simulink model "DCmotor_block"  (R2014b)
settings: Solver=ode23t  StartTime=0.0  StopTime=10  MaxStep=0.01  RelTol=1e-3
values from neighbouring files (symbols this model uses):
  Cv = 1.3*10^(-3) *10^(-3)*60/(2*pi)    (= 1.24140855612e-05)    [load_values.m]    (also in task6.m)
  J = 60 * 10^(-3) *10^(-4)    (= 6e-06)    [load_values.m]    (also in task6.m)
  kE = 4.555 *10^(-3)*60/(2*pi)    (= 0.043497045947)    [load_values.m]    (also in task6.m)
  kM = 43.5*10^(-3)    (= 0.0435)    [load_values.m]    (also in task6.m)
  L = [24.5, 19.6, 13.9, 13.1, 7   ] *10^(-3)    [load_values.m]    (also in task6.m = 0.00011)
  R = 1.45    [load_values.m]    (also in task6.m)
undefined symbols (not defined in the file or in its folder): MH
settings Model: Creator=Davide  LastModifiedBy=davidebo
settings DebuggingCC: SolverPrmCheckMsg=none

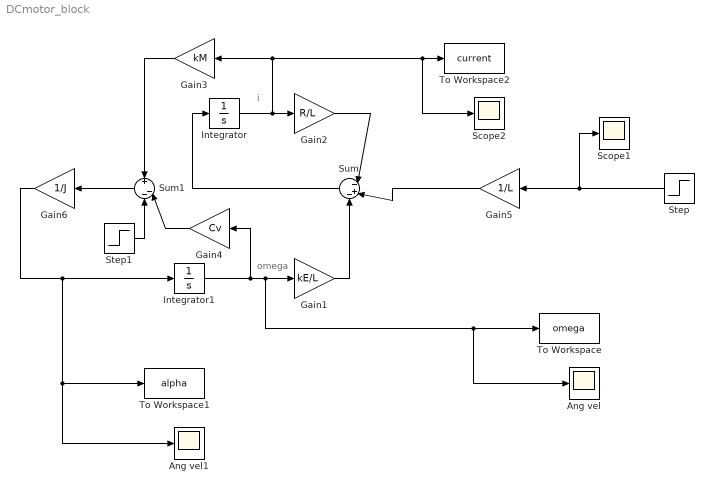
== system DCmotor_block ==
  note: omega
  note: i
  Ang vel : Scope
      settings: TimeRange=10
  Ang vel1 : Scope
      settings: TimeRange=10  SaveName=ScopeData2
  Gain1 : Gain  Gain=kE/L
  Gain2 : Gain  Gain=R/L
  Gain3 : Gain  Gain=kM
  Gain4 : Gain  Gain=Cv
  Gain5 : Gain  Gain=1/L
  Gain6 : Gain  Gain=1/J
  Integrator : Integrator
  Integrator1 : Integrator
  Scope1 : Scope
      settings: TimeRange=10
  Scope2 : Scope
      settings: TimeRange=10  SaveName=ScopeData3
  Step : Step  After=24  SampleTime=0
  Step1 : Step  Time=2  After=MH  SampleTime=0
  Sum : Sum  Inputs=|-+-
  Sum1 : Sum  Inputs=+|--
  To Workspace : ToWorkspace  VariableName=omega  SaveFormat=Timeseries  SampleTime=-1
  To Workspace1 : ToWorkspace  VariableName=alpha  SaveFormat=Timeseries  SampleTime=-1
  To Workspace2 : ToWorkspace  VariableName=current  SaveFormat=Timeseries  SampleTime=-1
  wires:
  Integrator/1 -> Scope2/1, To Workspace2/1, Gain3/1, Gain2/1
  Integrator1/1 -> Gain4/1, Ang vel/1, To Workspace/1, Gain1/1
  Gain2/1 -> Sum/1
  Sum/1 -> Integrator/1
  Gain1/1 -> Sum/3
  Gain3/1 -> Sum1/1
  Gain4/1 -> Sum1/2
  Gain5/1 -> Sum/2
  Sum1/1 -> Gain6/1
  Gain6/1 -> To Workspace1/1, Ang vel1/1, Integrator1/1
  Step1/1 -> Sum1/3
  Step/1 -> Scope1/1, Gain5/1
